simulink model "debugFT"  (Simulink 8.6)
settings: Solver=FixedStepDiscrete  StartTime=0.0  StopTime=inf  FixedStep=0.01  RelTol=1e-3
InitFcn:
  | ROBOT_DOF=23;
libraries: WBToolboxLibrary x13
settings Model: Creator=DanielePucci  LastModifiedBy=DanielePucci
settings DataIOCC: SaveFormat=Dataset  SignalLoggingSaveFormat=Dataset
settings OptimizationCC: ExpressionDepthLimit=128
settings DebuggingCC: UnderspecifiedInitializationDetection=Simplified  MergeDetectMultiDrivingBlocksExec=error  SolverPrmCheckMsg=none  FcnCallInpInsideContextMsg=EnableAllAsError  StateNameClashWarn=none
settings HardwareCC: ProdBitPerPointer=64  ProdLargestAtomicFloat=Float  ProdIntDivRoundTo=Zero  ProdEndianess=LittleEndian  ProdWordSize=64  ProdHWDeviceType=Intel->x86-64 (Windows64)
settings GRTTargetCC: GeneratePreprocessorConditionals=Use local settings  CombineOutputUpdateFcns=on  GRTInterface=off
settings ConfigComp: CovModelRefEnable=off

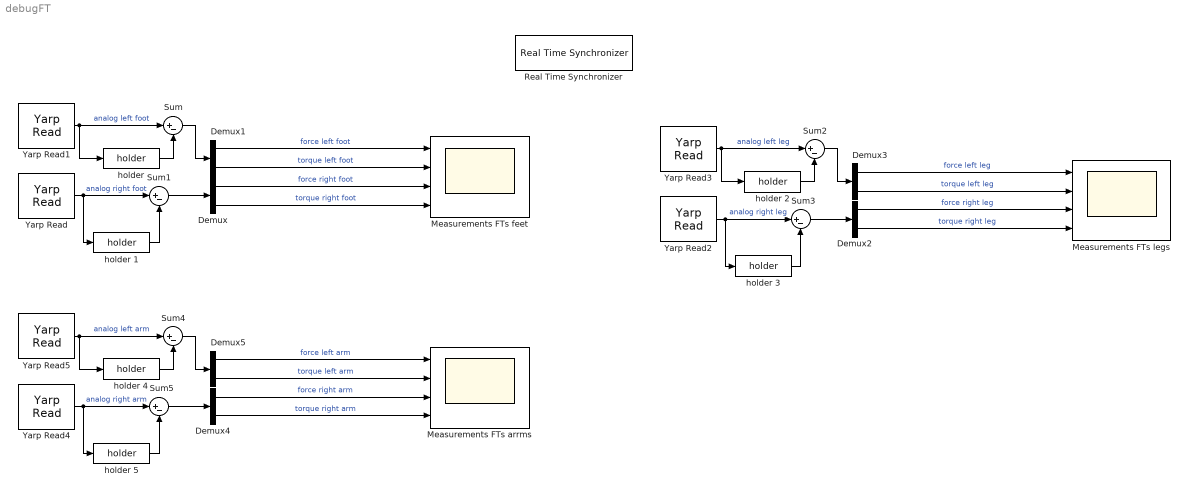
== system debugFT ==
  Demux{,1..5} (6 alike) : Demux  Outputs=2
  Measurements FTs arrms : Scope  NumInputPorts=4
  Measurements FTs feet : Scope  NumInputPorts=4
  Measurements FTs legs : Scope  NumInputPorts=4
  Real Time Synchronizer : WBToolboxLibrary/Utilities/Real Time Synchronizer  period=0.01
  Sum{,1..5} (6 alike) : Sum  Inputs=|+-
  Yarp Read : WBToolboxLibrary/Utilities/Yarp Read  portName='/icub/right_foot/analog:o'  signalSize=6  blocking=off  timestamp=off  autoconnect=on  errorOnConnection=off
  Yarp Read1 : WBToolboxLibrary/Utilities/Yarp Read  portName='/icub/left_foot/analog:o'  signalSize=6  blocking=off  timestamp=off  autoconnect=on  errorOnConnection=off
  Yarp Read2 : WBToolboxLibrary/Utilities/Yarp Read  portName='/icub/right_leg/analog:o'  signalSize=6  blocking=off  timestamp=off  autoconnect=on  errorOnConnection=off
  Yarp Read3 : WBToolboxLibrary/Utilities/Yarp Read  portName='/icub/left_leg/analog:o'  signalSize=6  blocking=off  timestamp=off  autoconnect=on  errorOnConnection=off
  Yarp Read4 : WBToolboxLibrary/Utilities/Yarp Read  portName='/icub/right_arm/analog:o'  signalSize=6  blocking=off  timestamp=off  autoconnect=on  errorOnConnection=off
  Yarp Read5 : WBToolboxLibrary/Utilities/Yarp Read  portName='/icub/left_arm/analog:o'  signalSize=6  blocking=off  timestamp=off  autoconnect=on  errorOnConnection=off
  holder {,1..5} (6 alike) : WBToolboxLibrary/Utilities/holder 
  wires:
  Yarp Read/1 -> holder 1/1, Sum1/1  "analog right foot"
  Demux/1 -> Measurements FTs feet/3  "force right foot"
  Demux/2 -> Measurements FTs feet/4  "torque right foot"
  Yarp Read1/1 -> "holder "/1, Sum/1  "analog left foot"
  Demux1/1 -> Measurements FTs feet/1  "force left foot"
  Demux1/2 -> Measurements FTs feet/2  "torque left foot"
  "holder "/1 -> Sum/2
  Sum/1 -> Demux1/1
  holder 1/1 -> Sum1/2
  Sum1/1 -> Demux/1
  Yarp Read2/1 -> holder 3/1, Sum3/1  "analog right leg"
  Demux2/1 -> Measurements FTs legs/3  "force right leg"
  Demux2/2 -> Measurements FTs legs/4  "torque right leg"
  Yarp Read3/1 -> holder 2/1, Sum2/1  "analog left leg"
  Demux3/1 -> Measurements FTs legs/1  "force left leg"
  Demux3/2 -> Measurements FTs legs/2  "torque left leg"
  holder 2/1 -> Sum2/2
  Sum2/1 -> Demux3/1
  holder 3/1 -> Sum3/2
  Sum3/1 -> Demux2/1
  Yarp Read4/1 -> holder 5/1, Sum5/1  "analog right arm"
  Demux4/1 -> Measurements FTs arrms/3  "force right arm"
  Demux4/2 -> Measurements FTs arrms/4  "torque right arm"
  Yarp Read5/1 -> holder 4/1, Sum4/1  "analog left arm"
  Demux5/1 -> Measurements FTs arrms/1  "force left arm"
  Demux5/2 -> Measurements FTs arrms/2  "torque left arm"
  holder 4/1 -> Sum4/2
  Sum4/1 -> Demux5/1
  holder 5/1 -> Sum5/2
  Sum5/1 -> Demux4/1
